simulink model "modelHandMuscleSystem"  (R2022b)
settings: Solver=ode4  StartTime=0.0  StopTime=4  FixedStep=0.001  RelTol=1e-3
model workspace (MAT data in the model file):
  aGain = 0.851191060499
  bGain = 1.702382121
  emgData.time = [0 0.001 0.002 0.003 0.004 0.005 0.006 0.007 0.008 0.009 0.01 0.011 ... (4001 elements, 4001x1)]
  emgData.signals.values = [2.43787182693e-05 2.43787182693e-05 2.43787182693e-05 2.43787182693e-05 2.43787182693e-05 2.43787182693e-05 2.43787102456e-05 2.43787015582e-05 2.43786922433e-05 2.43786822091e-05 2.43786715544e-05 2.43786601932e-05 ... (4001 elements, 4001x1)]
  spP.time = [0 0.001 0.002 0.003 0.004 0.005 0.006 0.007 0.008 0.009 0.01 0.011 ... (4001 elements, 4001x1)]
  spP.signals.values = [0 0 0 0 0 0 0 0 0 0 0 0 ... (4001 elements, 4001x1)]
libraries: dspsigops x2, simulink x1
settings Model: Creator=funato  LastModifiedBy=funato
settings OptimizationCC: ReuseModelBlockBuffer=on
settings ModelReferenceCC: EnableRefExpFcnMdlSchedulingChecks=on

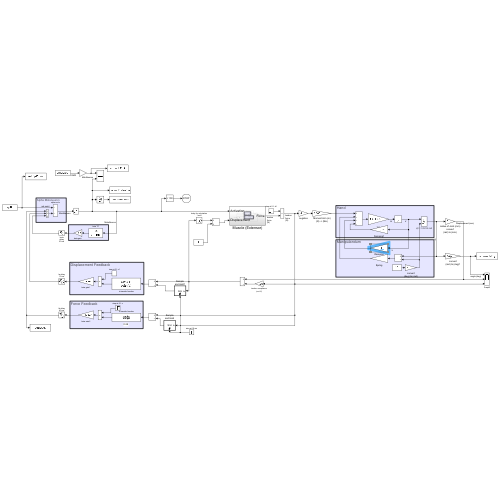
[thumbnail: Simulink's stored preview of the top-level diagram]
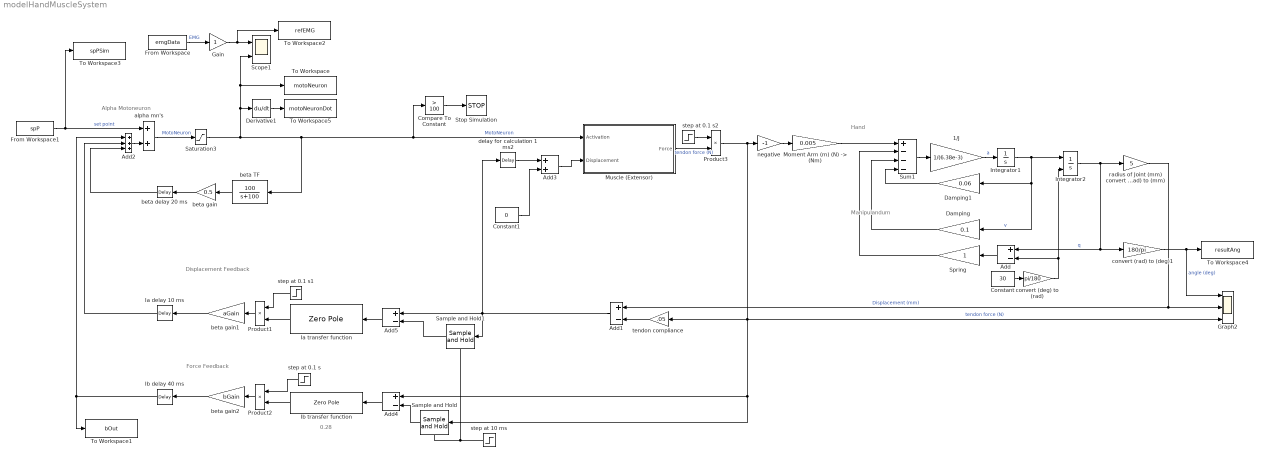
== system modelHandMuscleSystem ==
  note: Manipulandum
  note: Hand
  note: 0.28
  note: Displacement Feedback
  note: Force Feedback
  note: Alpha Motoneuron
  "1/J " : Gain  Gain=1/(6.38e-3)  SaturateOnIntegerOverflow=on  OutDataTypeStr=Inherit: Same as input  ParamDataTypeStr=Inherit: Same as input
  Add{,1,4..5} (4 alike) : Sum  Inputs=+-
  Add2 : Sum  Inputs=+++
  Add3 : Sum
  Compare To Constant : simulink/Logic and Bit Operations/Compare To Constant  relop=>  const=100  OutDataTypeStr=boolean
  Constant : Constant  Value=30
  Constant1 : Constant  Value=0
  Damping : Gain  Gain=0.1  SaturateOnIntegerOverflow=on  OutDataTypeStr=Inherit: Same as input  ParamDataTypeStr=Inherit: Same as input
  Damping1 : Gain  Gain=0.06  SaturateOnIntegerOverflow=on  OutDataTypeStr=Inherit: Same as input  ParamDataTypeStr=Inherit: Same as input
  Derivative1 : Derivative
  From Workspace : FromWorkspace  VariableName=emgData
  From Workspace1 : FromWorkspace  VariableName=spP
  Gain : Gain
  Graph2 : Scope  NumInputPorts=3
  Ia delay 10 ms : TransportDelay  DelayTime=.01
  Ia transfer function : ZeroPole  Zeros=[0; -.4; -4; -44]  Poles=[-.04; -.8; -100; -100]
  Ib delay 40 ms : TransportDelay  DelayTime=0.04
  Ib transfer function : ZeroPole  Zeros=[-.15; -1.5; -16]  Poles=[-.2; -2; -37]  Gain=[0.28]
  Integrator1 : Integrator
  Integrator2 : Integrator  InitialConditionSource=external  InitialCondition=0.5236
      settings: AttributesFormatString=q0 = %<InitialCondition> rad
  "Moment Arm (m) (N) -> (Nm)" : Gain  Gain=0.005
  Muscle (Extensor) : Subsystem
  Product1 : Product  InputSameDT=on  RndMeth=Zero  SaturateOnIntegerOverflow=on  OutDataTypeStr=Inherit: Same as first input
  Product2 : Product  InputSameDT=on  RndMeth=Zero  SaturateOnIntegerOverflow=on  OutDataTypeStr=Inherit: Same as first input
  Product3 : Product  InputSameDT=on  RndMeth=Zero  SaturateOnIntegerOverflow=on  OutDataTypeStr=Inherit: Same as first input
  Sample and Hold : dspsigops/Sample and Hold  trig=Rising edge  initCond=0  latchinput=off
  Sample and Hold1 : dspsigops/Sample and Hold  trig=Rising edge  initCond=0  latchinput=off
  Saturation3 : Saturate  UpperLimit=inf  LowerLimit=0
  Scope1 : Scope  NumInputPorts=2
  Spring : Gain  SaturateOnIntegerOverflow=on  OutDataTypeStr=Inherit: Same as input  ParamDataTypeStr=Inherit: Same as input
  Stop Simulation : Stop
  Sum1 : Sum  Inputs=+---  InputSameDT=on  SaturateOnIntegerOverflow=on  OutDataTypeStr=Inherit: Same as first input
  To Workspace : ToWorkspace  VariableName=motoNeuron  SaveFormat=Timeseries  SampleTime=-1
  To Workspace1 : ToWorkspace  VariableName=bOut  SaveFormat=Timeseries  SampleTime=-1
  To Workspace2 : ToWorkspace  VariableName=refEMG  SaveFormat=Timeseries  SampleTime=-1
  To Workspace3 : ToWorkspace  VariableName=spPSim  SaveFormat=Timeseries  SampleTime=-1
  To Workspace4 : ToWorkspace  VariableName=resultAng  SaveFormat=Timeseries  SampleTime=-1
  To Workspace5 : ToWorkspace  VariableName=motoNeuronDot  SaveFormat=Timeseries  SampleTime=-1
  alpha mn's : Sum  InputSameDT=on  SaturateOnIntegerOverflow=on  OutDataTypeStr=Inherit: Same as first input
  beta delay 20 ms : TransportDelay  DelayTime=.02
  beta TF : TransferFcn  Numerator=[100]  Denominator=[1 100]
  beta gain : Gain  Gain=0.5  SaturateOnIntegerOverflow=on  OutDataTypeStr=Inherit: Same as input  ParamDataTypeStr=Inherit: Same as input
  beta gain1 : Gain  Gain=aGain  SaturateOnIntegerOverflow=on  OutDataTypeStr=Inherit: Same as input  ParamDataTypeStr=Inherit: Same as input
  beta gain2 : Gain  Gain=bGain  SaturateOnIntegerOverflow=on  OutDataTypeStr=Inherit: Same as input  ParamDataTypeStr=Inherit: Same as input
  convert (deg) to (rad) : Gain  Gain=pi/180
  convert (rad) to (deg)1 : Gain  Gain=180/pi
  delay for calculation 1 ms2 : TransportDelay  DelayTime=.001  InitialOutput=2.6180
  negative : Gain  Gain=-1
  radius of Joint (mm) convert (rad) to (mm) : Gain  Gain=5
  step at 0.1 s : Step  Time=0.1  SampleTime=0.001
  step at 0.1 s1 : Step  Time=0.1  SampleTime=0.001
  step at 0.1 s2 : Step  Time=0.01  SampleTime=0.001
  step at 10 ms : Step  Time=0.02  SampleTime=0.001
  tendon compliance : Gain  Gain=.05  SaturateOnIntegerOverflow=on  OutDataTypeStr=Inherit: Same as input  ParamDataTypeStr=Inherit: Same as input
      settings: AttributesFormatString=(mm/N)
  wires:
  "1/J "/1 -> Integrator1/1  "a"
  Sum1/1 -> "1/J "/1
  "Moment Arm (m) (N) -> (Nm)"/1 -> Sum1/1
  negative/1 -> "Moment Arm (m) (N) -> (Nm)"/1
  Add1/1 -> Sample and Hold1/1, delay for calculation 1 ms2/1, Add5/1
  Spring/1 -> Sum1/2
  Damping/1 -> Sum1/3
  convert (rad) to (deg)1/1 -> To Workspace4/1, Graph2/1  "angle (deg)"
  Integrator2/1 -> radius of Joint (mm) convert (rad) to (mm)/1, Add/1, convert (rad) to (deg)1/1  "q"
  Ib transfer function/1 -> Product2/2
  beta gain2/1 -> Ib delay 40 ms/1
  tendon compliance/1 -> Add1/2
  step at 0.1 s/1 -> Product2/1
  Product2/1 -> beta gain2/1
  beta gain1/1 -> Ia delay 10 ms/1
  Add2/1 -> alpha mn's/2
  beta delay 20 ms/1 -> Add2/3
  Ib delay 40 ms/1 -> To Workspace1/1, Add2/1
  beta gain/1 -> beta delay 20 ms/1
  beta TF/1 -> beta gain/1
  radius of Joint (mm) convert (rad) to (mm)/1 -> Graph2/2, Add1/1  "Displacement (mm)"
  Product1/1 -> beta gain1/1
  Ia transfer function/1 -> Product1/2
  step at 0.1 s1/1 -> Product1/1
  Add/1 -> Spring/1
  Product3/1 -> tendon compliance/1, Add4/1, Sample and Hold/1, Graph2/3, negative/1  "tendon force (N)"
  step at 10 ms/1 -> Sample and Hold/Trigger, Sample and Hold1/Trigger
  Sample and Hold/1 -> Add4/2
  Add4/1 -> Ib transfer function/1
  Add5/1 -> Ia transfer function/1
  convert (deg) to (rad)/1 -> Integrator2/2, Add/2
  Sample and Hold1/1 -> Add5/2
  From Workspace1/1 -> alpha mn's/1, To Workspace3/1  "set point"
  Gain/1 -> To Workspace2/1, Scope1/1
  Saturation3/1 -> Derivative1/1, Scope1/2, To Workspace/1, Muscle (Extensor)/1(Activation), Compare To Constant/1, beta TF/1  "MotoNeuron"
  From Workspace/1 -> Gain/1  "EMG"
  Compare To Constant/1 -> Stop Simulation/1
  Damping1/1 -> Sum1/4
  Integrator1/1 -> Damping/1, Damping1/1, Integrator2/1  "v"
  Ia delay 10 ms/1 -> Add2/2
  step at 0.1 s2/1 -> Product3/1
  Muscle (Extensor)/1(Force) -> Product3/2  "tendon force (N)"
  Constant/1 -> convert (deg) to (rad)/1
  Add3/1 -> Muscle (Extensor)/2(Displacement)
  delay for calculation 1 ms2/1 -> Add3/1
  Constant1/1 -> Add3/2
  alpha mn's/1 -> Saturation3/1  "MotoNeuron"
  Derivative1/1 -> To Workspace5/1

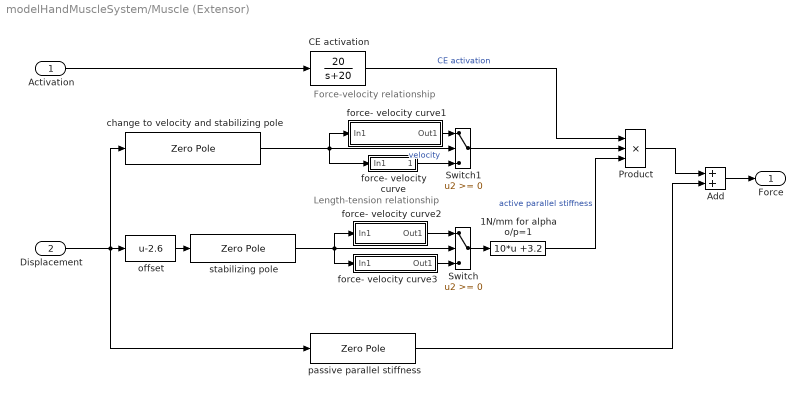
== system modelHandMuscleSystem/Muscle (Extensor) ==
  note: Length-tension relationship
  note: Force-velocity relationship
  Activation : Inport
  Displacement : Inport  Port=2
  1N/mm for alpha o/p=1 : Fcn  Expr=10*u +3.2
  Add : Sum
  CE activation : TransferFcn  Numerator=[20]  Denominator=[1 20]
      settings: AttributesFormatString=|
      | Low-pass Filter
      | cutoff: 20 (rad/s)=3.2Hz
  Product : Product  Inputs=3  InputSameDT=on  RndMeth=Zero  SaturateOnIntegerOverflow=on  OutDataTypeStr=Inherit: Same as first input
  Switch : Switch
  Switch1 : Switch
  change to velocity and stabilizing pole : ZeroPole  Zeros=[0]  Poles=[-500,-500]  Gain=[1500]
  force- velocity curve : Subsystem
      mask Display: disp('1/(1-u)')
  force- velocity curve1 : Subsystem
      mask Display: disp('1+.5(1-exp(-1.5u))')
  force- velocity curve2 : Subsystem
      mask Display: disp('1-exp(-.15u)')
  force- velocity curve3 : Subsystem
      mask Display: disp('-1+exp(.15u)')
  offset : Fcn  Expr=u-2.6
  passive parallel stiffness : ZeroPole  Zeros=[-25]  Poles=[-500]  Gain=[5]
      settings: AttributesFormatString=.25N/mm
  stabilizing pole : ZeroPole  Zeros=[ ]  Poles=[-500]  Gain=[500]
      settings: AttributesFormatString=|
      | Low-pass Filter
      | cutoff: %<Gain>(rad/s)
  Force : Outport
  wires:
  CE activation/1 -> Product/1  "CE activation"
  passive parallel stiffness/1 -> Add/2
  Activation/1 -> CE activation/1
  Product/1 -> Add/1
  change to velocity and stabilizing pole/1 -> force- velocity curve/1(In1), Switch1/2, force- velocity curve1/1(In1)  "velocity"
  Switch/1 -> 1N/mm for alpha o/p=1/1
  Switch1/1 -> Product/2
  stabilizing pole/1 -> force- velocity curve3/1(In1), Switch/2, force- velocity curve2/1(In1)
  force- velocity curve1/1(Out1) -> Switch1/1
  force- velocity curve/1(Out1) -> Switch1/3
  1N/mm for alpha o/p=1/1 -> Product/3  "active parallel stiffness"
  offset/1 -> stabilizing pole/1
  force- velocity curve3/1(Out1) -> Switch/3
  force- velocity curve2/1(Out1) -> Switch/1
  Add/1 -> Force/1
  Displacement/1 -> passive parallel stiffness/1, change to velocity and stabilizing pole/1, offset/1

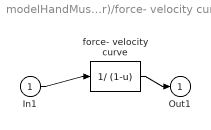
== system modelHandMuscleSystem/Muscle (Extensor)/force- velocity curve ==
  In1 : Inport
  force- velocity curve : Fcn  Expr=1/ (1-u)
  Out1 : Outport
  wires:
  In1/1 -> force- velocity curve/1
  force- velocity curve/1 -> Out1/1

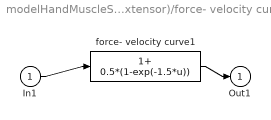
== system modelHandMuscleSystem/Muscle (Extensor)/force- velocity curve1 ==
  In1 : Inport
  force- velocity curve1 : Fcn  Expr=1+ 0.5*(1-exp(-1.5*u))
  Out1 : Outport
  wires:
  In1/1 -> force- velocity curve1/1
  force- velocity curve1/1 -> Out1/1

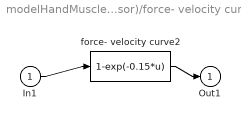
== system modelHandMuscleSystem/Muscle (Extensor)/force- velocity curve2 ==
  In1 : Inport
  force- velocity curve2 : Fcn  Expr=1-exp(-0.15*u)
  Out1 : Outport
  wires:
  In1/1 -> force- velocity curve2/1
  force- velocity curve2/1 -> Out1/1

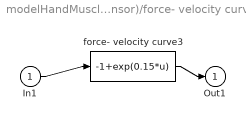
== system modelHandMuscleSystem/Muscle (Extensor)/force- velocity curve3 ==
  In1 : Inport
  force- velocity curve3 : Fcn  Expr=-1+exp(0.15*u)
  Out1 : Outport
  wires:
  In1/1 -> force- velocity curve3/1
  force- velocity curve3/1 -> Out1/1
